simulink model "realtime_Euler_Pos_state_space"  (R2024b)
settings: Solver=FixedStepDiscrete  StartTime=0.0  StopTime=10  FixedStep=0.001  RelTol=1e-3
values from neighbouring files (symbols this model uses):
  Gamma_o = Bo * T    [Pos_state_space.m]
  Ho = Co    [Pos_state_space.m]
  Jo = Do    [Pos_state_space.m]
  K = acker(A,B,poles)    [Pos_state_space.m]    (also in code_ali.m)
  Nu = Ans(3,1)    [Pos_state_space.m]    (also in code_ali.m)
  Nx = Ans(1:2,1)    [Pos_state_space.m]    (also in code_ali.m)
  Phi_o = 1 + Ao * T    [Pos_state_space.m]
  T = 0.001*50    (= 0.05)    [Pos_state_space.m]
undefined symbols (not defined in the file or in its folder): National_Instruments, PCI, rpm2rads
libraries: sldrtlib x2
settings Model: SimulationMode=external  ExtModeTrigDuration=1000001  Creator=galeazzolu  LastModifiedBy=galeazzolu
settings DataIOCC: ReturnWorkspaceOutputs=off
settings HardwareCC: ProdBitPerLong=64  ProdHWDeviceType=Intel->x86-64 (Linux 64)
settings RTWCC: Description=Simulink Desktop Real-Time  SystemTargetFile=sldrt.tlc  TemplateMakefile=sldrt.tmf  RTWCompilerOptimization=on
settings CodeAppCC: MaxIdLength=95
settings SimulinkDesktopRealTimeCC: TargetLibSuffix=_sldrt.a  TargetPreCompLibLocation=C:\Program Files\MATLAB\R2024b\toolbox\sldrt\lib\win64  ParMdlRefBuildCompliant=on

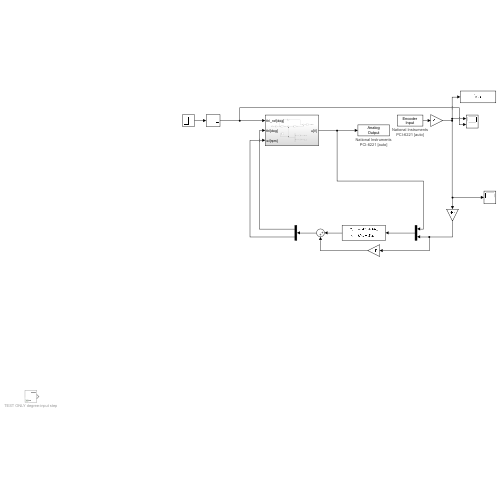
[thumbnail: Simulink's stored preview of the top-level diagram]
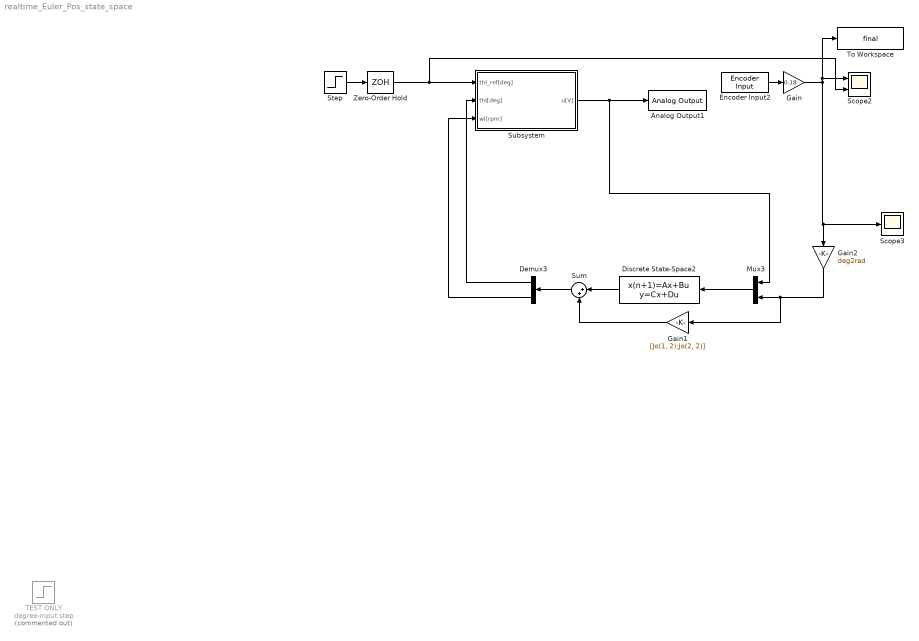
== system realtime_Euler_Pos_state_space ==
  Analog Output1 : sldrtlib/Analog Output  SampleTime=T  MaxMissedTicks=10  ShowMissedTicks=off  YieldWhenWaiting=off  DrvName=National_Instruments/PCI-6221  DrvAddress=4294967295  DrvOptions=[0 0 0 2 0]  Channels=1  RangeMode=1  VoltRange=1  InitialValue=0  FinalValue=0
      settings: AttributesFormatString=National Instruments\nPCI-6221 [auto]
  Demux3 : Demux  Outputs=2
  Discrete State-Space2 : DiscreteStateSpace  A=Phi_o  B=Gamma_o  C=Ho  D=[0,0;0,0]  SampleTime=T
  Encoder Input2 : sldrtlib/Encoder Input  SampleTime=T  MaxMissedTicks=10  ShowMissedTicks=off  YieldWhenWaiting=off  DrvName=National_Instruments/PCI-6221  DrvAddress=4294967295  DrvOptions=[0 0 0 2 0]  Channels=1  QuadMode=3  IndexPulse=1  InputFilter=Inf  DataType=1
      settings: AttributesFormatString=National Instruments\nPCI-6221 [auto]
  Gain : Gain  Gain=0.18
  Gain1 : Gain  Gain=[Jo(1, 2);Jo(2, 2)]
  Gain2 : Gain  Gain=deg2rad
  Mux3 : Mux  Inputs=2
  Scope2 : Scope  NumInputPorts=2
  Scope3 : Scope
  Step : Step  After=50  SampleTime=0
  Subsystem : Subsystem
  Sum : Sum  Inputs=|++
  TEST ONLY degree-input step : Step  Commented=on  After=360  SampleTime=0
  To Workspace : ToWorkspace  VariableName=final  SaveFormat=Structure With Time  SampleTime=-1
  Zero-Order Hold : ZeroOrderHold  SampleTime=T
  wires:
  Gain/1 -> To Workspace/1, Scope2/1, Scope3/1, Gain2/1
  Encoder Input2/1 -> Gain/1
  Zero-Order Hold/1 -> Scope2/2, Subsystem/1(thl_ref[deg])
  Step/1 -> Zero-Order Hold/1
  Gain2/1 -> Mux3/2, Gain1/1
  Demux3/1 -> Subsystem/2(thl[deg])
  Gain1/1 -> Sum/2
  Discrete State-Space2/1 -> Sum/1
  Mux3/1 -> Discrete State-Space2/1
  Subsystem/1(u[V]) -> Mux3/1, Analog Output1/1
  Demux3/2 -> Subsystem/3(wl[rpm])
  Sum/1 -> Demux3/1

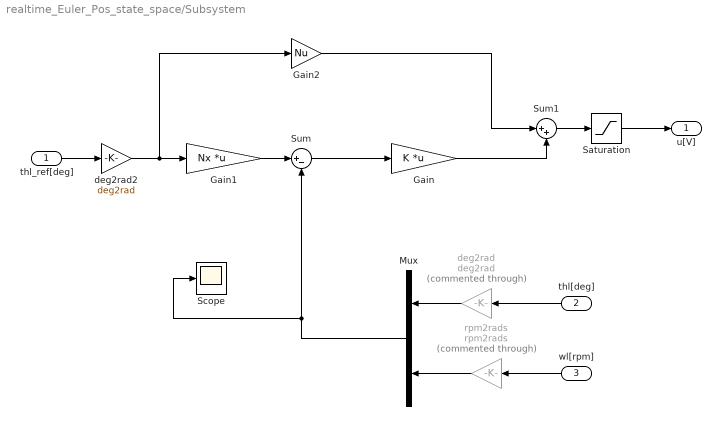
== system realtime_Euler_Pos_state_space/Subsystem ==
  thl_ref[deg] : Inport
  thl[deg] : Inport  Port=2
  wl[rpm] : Inport  Port=3
  Gain : Gain  Gain=K  Multiplication=Matrix(K*u)
  Gain1 : Gain  Gain=Nx  Multiplication=Matrix(K*u)
  Gain2 : Gain  Gain=Nu
  Mux : Mux  Inputs=2
  Saturation : Saturate  UpperLimit=12  LowerLimit=-12
  Scope : Scope
  Sum : Sum  Inputs=|+-
  Sum1 : Sum  Inputs=|++
  deg2rad : Gain  Commented=through  Gain=deg2rad
  deg2rad2 : Gain  Gain=deg2rad
  rpm2rads : Gain  Commented=through  Gain=rpm2rads
  u[V] : Outport
  wires:
  thl[deg]/1 -> deg2rad/1
  wl[rpm]/1 -> rpm2rads/1
  deg2rad/1 -> Mux/1
  rpm2rads/1 -> Mux/2
  Mux/1 -> Sum/2, Scope/1
  Sum/1 -> Gain/1
  Gain1/1 -> Sum/1
  thl_ref[deg]/1 -> deg2rad2/1
  deg2rad2/1 -> Gain1/1, Gain2/1
  Gain2/1 -> Sum1/1
  Gain/1 -> Sum1/2
  Sum1/1 -> Saturation/1
  Saturation/1 -> u[V]/1
